simulink model "CL"  (R2017a)
settings: Solver=VariableStepAuto  StartTime=0.0  StopTime=50  RelTol=1e-3
values from neighbouring files (symbols this model uses):
  A = [0 1 0 0;-k/j2 -b/j2 k/j2 b/j2;0 0 0 01;k/j1 b/j1 -k/j1 -b/j1]    [sys1.m]
  B = [b -b;-b b]    [dynamic_using_Nemark_controller.m]    (also in sys1.m = [0;0;0;1/j1])
  C = [1 0 0 0]    [sys1.m]
  D = zeros(1,1)    [sys1.m]
settings Model: Creator=ASUS  LastModifiedBy=ASUS

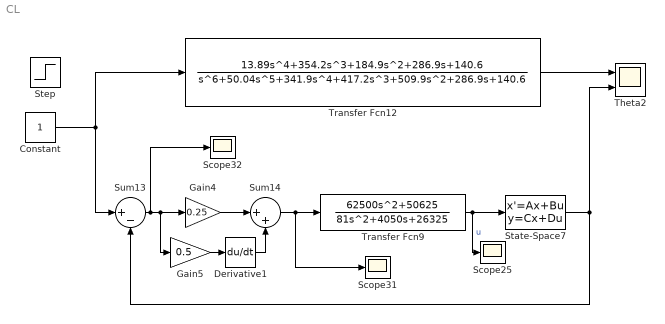
== system CL ==
  Constant : Constant
  Derivative1 : Derivative
  Gain4 : Gain  Gain=0.25
  Gain5 : Gain  Gain=0.5
  Scope25 : Scope
  Scope31 : Scope
  Scope32 : Scope
  State-Space7 : StateSpace  A=A  B=B  C=C  D=D  X0=[0 0 0 0]
  Step : Step  SampleTime=0
  Sum13 : Sum  Inputs=|+-
  Sum14 : Sum  Inputs=|++
  Theta2 : Scope  NumInputPorts=2
  Transfer Fcn12 : TransferFcn  Numerator=[13.89 354.2 184.9 286.9 140.6]  Denominator=[1 50.04 341.9 417.2 509.9 286.9 140.6]
  Transfer Fcn9 : TransferFcn  Numerator=[62500 0 50625]  Denominator=[81 4050 26325]
  wires:
  Constant/1 -> Transfer Fcn12/1, Sum13/1
  Transfer Fcn12/1 -> Theta2/1
  Sum13/1 -> Scope32/1, Gain5/1, Gain4/1
  Sum14/1 -> Scope31/1, Transfer Fcn9/1
  Derivative1/1 -> Sum14/2
  Gain5/1 -> Derivative1/1
  Transfer Fcn9/1 -> State-Space7/1, Scope25/1  "u"
  State-Space7/1 -> Theta2/2, Sum13/2
  Gain4/1 -> Sum14/1
